simulink model "Control_referencia"  (Simulink 9.0)
settings: Solver=VariableStepAuto  StartTime=0.0  StopTime=t  RelTol=1e-3
values from neighbouring files (symbols this model uses):
  k = -1.1735    [Ensayo_Steer_control.m]
  P = 50    [Ensayo_Steer_control.m]
  q0 = Ks*(1+T/(2*Tis))    (= -0.454196847039)    [Ensayo_Steer_control.m]
  q1 = Ks*(-1+T/(2*Tis))    (= 0.028121005539)    [Ensayo_Steer_control.m]
  qden_cp = [1 -1 0]    [Ensayo_Steer_control.m]
  qnum_cp = [q0p q1p q2p]    [Ensayo_Steer_control.m]
  T = 0.05    [Ensayo_Steer_control.m]
  t_p = 7    [Ensayo_Steer_control.m]
  tau = 0.0283    [Ensayo_Steer_control.m]
undefined symbols (not defined in the file or in its folder): DiscIntNeverNeededParam
settings Model: Creator=Francisco José Mañas  LastModifiedBy=Lab110PC3
settings DataIOCC: SaveFormat=Dataset
settings OptimizationCC: LifeSpan=auto
settings DebuggingCC: UnderspecifiedInitializationDetection=Simplified  MergeDetectMultiDrivingBlocksExec=error  SFUnexpectedBacktrackingDiag=error  SFNoUnconditionalDefaultTransitionDiag=error  SFExecutionAtInitializationDiag=warning
settings HardwareCC: ProdBitPerPointer=64  ProdBitPerSizeT=64  ProdBitPerPtrDiffT=64  ProdLargestAtomicFloat=Float  ProdIntDivRoundTo=Zero  ProdEndianess=LittleEndian  ProdWordSize=64  ProdHWDeviceType=Intel->x86-64 (Windows64)
settings ModelReferenceCC: PropagateSignalLabelsOutOfModel=on
settings GRTTargetCC: TargetLangStandard=C99 (ISO)
settings ConfigComp: CovMetricSettings=dwe  CovHtmlReporting=off  CovSaveCumulativeToWorkspaceVar=off  CovSaveSingleToWorkspaceVar=off  CovExternalEMLEnable=on

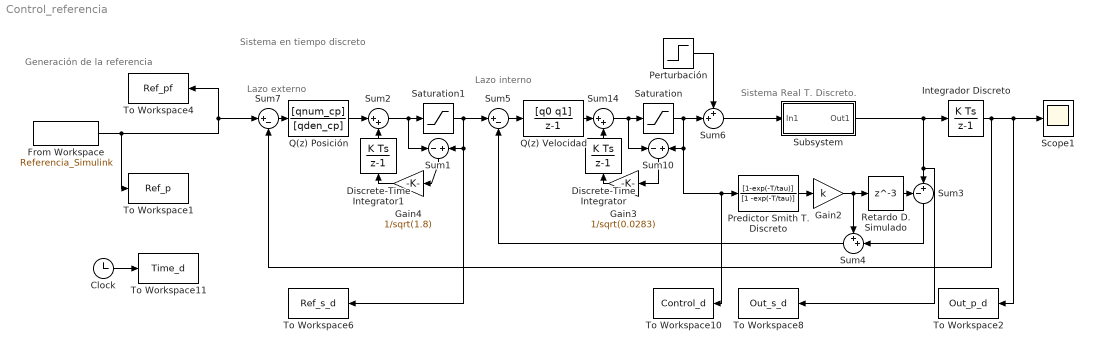
== system Control_referencia ==
  note: Sistema Real T. Discreto.
  note: Lazo externo
  note: Generación de la referencia
  note: Sistema en tiempo discreto
  note: Lazo interno
  Clock : Clock
  Discrete-Time Integrator : DiscreteIntegrator  InitialConditionSetting=State (most efficient)  SampleTime=-1  ICPrevOutput=DiscIntNeverNeededParam  ICPrevScaledInput=DiscIntNeverNeededParam
  Discrete-Time Integrator1 : DiscreteIntegrator  InitialConditionSetting=State (most efficient)  SampleTime=-1  ICPrevOutput=DiscIntNeverNeededParam  ICPrevScaledInput=DiscIntNeverNeededParam
  From Workspace : FromWorkspace  VariableName=Referencia_Simulink  SampleTime=T
  Gain2 : Gain  Gain=k
  Gain3 : Gain  Gain=1/sqrt(0.0283)
  Gain4 : Gain  Gain=1/sqrt(1.8)
  Integrador Discreto : DiscreteIntegrator  InitialConditionSetting=State (most efficient)  SampleTime=T  ICPrevOutput=DiscIntNeverNeededParam  ICPrevScaledInput=DiscIntNeverNeededParam
  Perturbación : Step  Time=t_p  After=P  SampleTime=0
  Predictor Smith T. Discreto : DiscreteTransferFcn  Numerator=[1-exp(-T/tau)]  Denominator=[1 -exp(-T/tau)]  SampleTime=T
  Q(z) Posición : DiscreteTransferFcn  Numerator=[qnum_cp]  Denominator=[qden_cp]  SampleTime=T
  Q(z) Velocidad : DiscreteTransferFcn  Numerator=[q0 q1]  Denominator=[1 -1]
  Retardo D. Simulado : Delay  DelayLength=3  SampleTime=T
  Saturation : Saturate  UpperLimit=254  LowerLimit=-254
  Saturation1 : Saturate  UpperLimit=1024  LowerLimit=-1024
  Scope1 : Scope
  Subsystem : Subsystem
  Sum1 : Sum  Inputs=-+
  Sum10 : Sum  Inputs=-+
  Sum14 : Sum  Inputs=|++
  Sum2 : Sum  Inputs=|++
  Sum3 : Sum  Inputs=-+|
  Sum4 : Sum  Inputs=++|
  Sum5 : Sum  Inputs=|+-
  Sum6 : Sum  Inputs=++|
  Sum7 : Sum  Inputs=|+-
  To Workspace1 : ToWorkspace  VariableName=Ref_p  SampleTime=T
  To Workspace10 : ToWorkspace  VariableName=Control_d  SampleTime=-1
  To Workspace11 : ToWorkspace  VariableName=Time_d  SampleTime=T
  To Workspace2 : ToWorkspace  VariableName=Out_p_d  SampleTime=T
  To Workspace4 : ToWorkspace  VariableName=Ref_pf  SampleTime=T
  To Workspace6 : ToWorkspace  VariableName=Ref_s_d  SampleTime=-1
  To Workspace8 : ToWorkspace  VariableName=Out_s_d  SampleTime=-1
  wires:
  Clock/1 -> To Workspace11/1
  Predictor Smith T. Discreto/1 -> Gain2/1
  Gain2/1 -> Retardo D. Simulado/1, Sum4/1
  Retardo D. Simulado/1 -> Sum3/1
  Sum3/1 -> Sum4/2
  Sum5/1 -> Q(z) Velocidad/1
  Sum4/1 -> Sum5/2
  Q(z) Posición/1 -> Sum2/1
  Sum7/1 -> Q(z) Posición/1
  Saturation/1 -> Sum6/2, Sum10/2, Predictor Smith T. Discreto/1, To Workspace10/1
  From Workspace/1 -> To Workspace4/1, Sum7/1, To Workspace1/1
  Integrador Discreto/1 -> To Workspace2/1, Scope1/1, Sum7/2
  Sum14/1 -> Sum10/1, Saturation/1
  Discrete-Time Integrator/1 -> Sum14/2
  Gain3/1 -> Discrete-Time Integrator/1
  Sum10/1 -> Gain3/1
  Q(z) Velocidad/1 -> Sum14/1
  Saturation1/1 -> To Workspace6/1, Sum1/2, Sum5/1
  Sum2/1 -> Sum1/1, Saturation1/1
  Discrete-Time Integrator1/1 -> Sum2/2
  Sum1/1 -> Gain4/1
  Gain4/1 -> Discrete-Time Integrator1/1
  Subsystem/1(Out1) -> To Workspace8/1, Sum3/2, Integrador Discreto/1
  Sum6/1 -> Subsystem/1(In1)
  Perturbación/1 -> Sum6/1

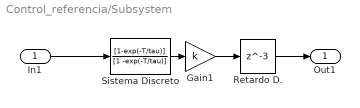
== system Control_referencia/Subsystem ==
  In1 : Inport
  Gain1 : Gain  Gain=k
  Retardo D. : Delay  DelayLength=3  SampleTime=T
  Sistema Discreto : DiscreteTransferFcn  Numerator=[1-exp(-T/tau)]  Denominator=[1 -exp(-T/tau)]  SampleTime=T
  Out1 : Outport
  wires:
  In1/1 -> Sistema Discreto/1
  Sistema Discreto/1 -> Gain1/1
  Retardo D./1 -> Out1/1
  Gain1/1 -> Retardo D./1
